simulink model "CDR_Basic_lib"  (R2012b)
settings: Solver=ode45  StartTime=0.0  StopTime=10.0  RelTol=1e-3
values from neighbouring files (symbols this model uses):
  Ts = 1/fbit/OSR    (= 0.01)    [init_pr_bb_cdr.m]
undefined symbols (not defined in the file): Fosc, Int_Divider, Tsymbol, VDD
libraries: simulink_extras x124, simulink x3
(part 1 of 2)
settings Model: ExtModeAutoUpdateStatusClock=off  Creator=Hemesh Yasotharan  LastModifiedBy=Tony
settings DataIOCC: SignalLoggingSaveFormat=ModelDataLogs
settings OptimizationCC: InitFltsAndDblsToZero=on
settings DebuggingCC: SaveWithParameterizedLinksMsg=none  FcnCallInpInsideContextMsg=UseLocalSettings  StrictBusMsg=Warning
settings GRTTargetCC: TargetFcnLib=ansi_tfl_tmw.mat  CombineOutputUpdateFcns=off  GRTInterface=on

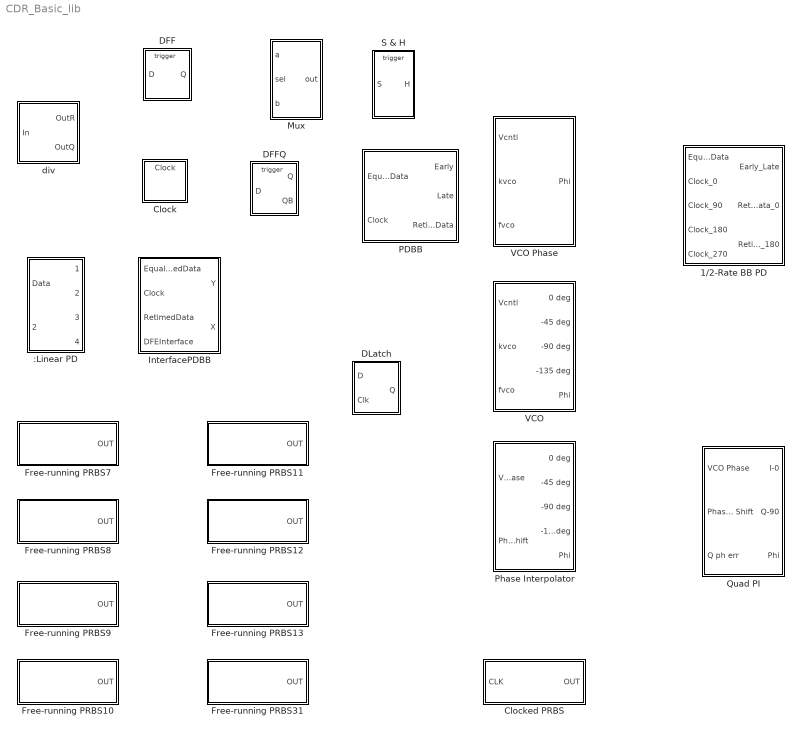
== system CDR_Basic_lib ==
  1/2-Rate BB PD : Subsystem  mask{VDD=1}
  :Linear PD : Subsystem  mask{VDD=VDD}
  Clock : Subsystem  mask{Period=0, PulseWidth=0}
      mask prompts: Period "Samples in one Period"; PulseWidth "Samples in the Pulse width"
  Clocked PRBS : Subsystem  mask{rst_time=0, X00=1, X01=1, X02=1, X03=1, X04=1, X05=1, X06=1, X07=1, X08=1, X09=1}
      mask prompts: rst_time "Reset time"; X00 "X00 [0,1]:"; X01 "X01 [0,1]:"; X02 "X02 [0,1]:"; X03 "X03 [0,1]:"; X04 "X04 [0,1]:"; X05 "X05 [0,1]:"; X06 "X06 [0,1]:"; X07 "X07 [0,1]:"; X08 "X08 [0,1]:"; X09 "X09 [0,1]:"
      mask help: Enter the initial state [0,1] below.
      mask Display: disp('PRBS_2^10')
  DFF : Subsystem  mask{DataHigh=1, DataLow=0, FF_Threshold=0.5}
      mask prompts: DataHigh "High Data Value"; DataLow "Low Data Value"; FF_Threshold "Flip-Flop Threshold"
  DFFQ : Subsystem  mask{DataHigh=1, DataLow=0, FF_Threshold=0.5}
      mask prompts: DataHigh "High Data Value"; DataLow "Low Data Value"; FF_Threshold "Flip-Flop Threshold"
  DLatch : Subsystem  mask{DataHigh=VDD, DataLow=0, L_Threshold=VDD/2}
      mask prompts: DataHigh "High Data Value"; DataLow "Low Data Value"; L_Threshold "Latch Threshold"
  Free-running PRBS10 : Subsystem  mask{sample_prd=Ts, symbol_prd=Tsymbol, X00=1, X01=1, X02=1, X03=1, X04=1, X05=1, X06=1, X07=1, X08=1, X09=1}
      mask prompts: sample_prd "Sample Time [s]:"; symbol_prd "Symbol Period [s]:"; X00 "X00 [0,1]:"; X01 "X01 [0,1]:"; X02 "X02 [0,1]:"; X03 "X03 [0,1]:"; X04 "X04 [0,1]:"; X05 "X05 [0,1]:"; X06 "X06 [0,1]:"; X07 "X07 [0,1]:"; X08 "X08 [0,1]:"; X09 "X09 [0,1]:"
      mask help: Enter the initial state [0,1] below.
      mask Display: disp('PRBS_2^10')
  Free-running PRBS11 : Subsystem  mask{sample_prd=Ts, symbol_prd=Tsymbol, X00=1, X01=1, X02=1, X03=1, X04=1, X05=1, X06=1, X07=1, X08=1, X09=1, X10=1}
      mask prompts: sample_prd "Sample Time [s]:"; symbol_prd "Symbol Period [s]:"; X00 "X00 [0,1]:"; X01 "X01 [0,1]:"; X02 "X02 [0,1]:"; X03 "X03 [0,1]:"; X04 "X04 [0,1]:"; X05 "X05 [0,1]:"; X06 "X06 [0,1]:"; X07 "X07 [0,1]:"; X08 "X08 [0,1]:"; X09 "X09 [0,1]:"; X10 "X10 [0,1]:"
      mask help: Enter the initial state [0,1] below.
      mask Display: disp('PRBS_2^11')
  Free-running PRBS12 : Subsystem  mask{sample_prd=Ts, symbol_prd=Tsymbol, X00=1, X01=1, X02=1, X03=1, X04=1, X05=1, X06=1, X07=1, X08=1, X09=1, X10=1, X11=1}
      mask prompts: sample_prd "Sample Time [s]:"; symbol_prd "Symbol Period [s]:"; X00 "X00 [0,1]:"; X01 "X01 [0,1]:"; X02 "X02 [0,1]:"; X03 "X03 [0,1]:"; X04 "X04 [0,1]:"; X05 "X05 [0,1]:"; X06 "X06 [0,1]:"; X07 "X07 [0,1]:"; X08 "X08 [0,1]:"; X09 "X09 [0,1]:"; X10 "X10 [0,1]:"; X11 "X11 [0,1]:"
      mask help: Enter the initial state [0,1] below.
      mask Display: disp('PRBS_2^12')
  Free-running PRBS13 : Subsystem  mask{sample_prd=Ts, symbol_prd=Tsymbol, X00=1, X01=1, X02=1, X03=1, X04=1, X05=1, X06=1, X07=1, X08=1, X09=1, X10=1, X11=1, X12=1}
      mask prompts: sample_prd "Sample Time [s]:"; symbol_prd "Symbol Period [s]:"; X00 "X00 [0,1]:"; X01 "X01 [0,1]:"; X02 "X02 [0,1]:"; X03 "X03 [0,1]:"; X04 "X04 [0,1]:"; X05 "X05 [0,1]:"; X06 "X06 [0,1]:"; X07 "X07 [0,1]:"; X08 "X08 [0,1]:"; X09 "X09 [0,1]:"; X10 "X10 [0,1]:"; X11 "X11 [0,1]:"; X12 "X12 [0,1]:"
      mask help: Enter the initial state [0,1] below.
      mask Display: disp('PRBS_2^13')
  Free-running PRBS31 : Subsystem  mask{sample_prd=Ts, symbol_prd=Tsymbol, X00=1, X01=1, X02=1, X03=1, X04=1, X05=1, X06=1, X07=1, X08=1, X09=1, X10=1, X11=1, X12=1, X13=1, X14=1, X15=1, X16=1, X17=1, X18=1, X19=1, X20=1, X21=1, X22=1, X23=1, X24=1, X25=1, X26=1, X27=1, X28=1, X29=1, X30=1}
      mask prompts: sample_prd "Sample Time [s]:"; symbol_prd "Symbol Period [s]:"; X00 "X00 [0,1]:"; X01 "X01 [0,1]:"; X02 "X02 [0,1]:"; X03 "X03 [0,1]:"; X04 "X04 [0,1]:"; X05 "X05 [0,1]:"; X06 "X06 [0,1]:"; X07 "X07 [0,1]:"; X08 "X08 [0,1]:"; X09 "X09 [0,1]:"; X10 "X10 [0,1]:"; X11 "X11 [0,1]:"; X12 "X12 [0,1]:"; X13 "X13 [0,1]:"; X14 "X14 [0,1]:"; X15 "X15 [0,1]:"; X16 "X16 [0,1]:"; X17 "X17 [0,1]:"; X18 "X18 [0,1]:"; X19 "X19 [0,1]:"; X20 "X20 [0,1]:"; X21 "X21 [0,1]:"; X22 "X22 [0,1]:"; X23 "X23 [0,1]:"; X24 "X24 [0,1]:"; X25 "X25 [0,1]:"; X26 "X26 [0,1]:"; X27 "X27 [0,1]:"; X28 "X28 [0,1]:"; X29 "X29 [0,1]:"; X30 "X30 [0,1]:"
      mask help: Enter the initial state [0,1] below.
      mask Display: disp('PRBS_2^31')
  Free-running PRBS7 : Subsystem  mask{sample_prd=Ts, symbol_prd=Tsymbol, X00=1, X01=1, X02=1, X03=1, X04=1, X05=1, X06=1}
      mask prompts: sample_prd "Sample Time [s]:"; symbol_prd "Symbol Period [s]:"; X00 "X00 [0,1]:"; X01 "X01 [0,1]:"; X02 "X02 [0,1]:"; X03 "X03 [0,1]:"; X04 "X04 [0,1]:"; X05 "X05 [0,1]:"; X06 "X06 [0,1]:"
      mask help: Enter the initial state [0,1] below.
      mask Display: disp('PRBS_2^7')
  Free-running PRBS8 : Subsystem  mask{sample_prd=Ts, symbol_prd=Tsymbol, X00=1, X01=1, X02=1, X03=1, X04=1, X05=1, X06=1, X07=1}
      mask prompts: sample_prd "Sample Time [s]:"; symbol_prd "Symbol Period [s]:"; X00 "X00 [0,1]:"; X01 "X01 [0,1]:"; X02 "X02 [0,1]:"; X03 "X03 [0,1]:"; X04 "X04 [0,1]:"; X05 "X05 [0,1]:"; X06 "X06 [0,1]:"; X07 "X07 [0,1]:"
      mask help: Enter the initial state [0,1] below.
      mask Display: disp('PRBS_2^8')
  Free-running PRBS9 : Subsystem  mask{sample_prd=Ts, symbol_prd=Tsymbol, X00=1, X01=1, X02=1, X03=1, X04=1, X05=1, X06=1, X07=1, X08=1}
      mask prompts: sample_prd "Sample Time [s]:"; symbol_prd "Symbol Period [s]:"; X00 "X00 [0,1]:"; X01 "X01 [0,1]:"; X02 "X02 [0,1]:"; X03 "X03 [0,1]:"; X04 "X04 [0,1]:"; X05 "X05 [0,1]:"; X06 "X06 [0,1]:"; X07 "X07 [0,1]:"; X08 "X08 [0,1]:"
      mask help: Enter the initial state [0,1] below.
      mask Display: disp('PRBS_2^9')
  InterfacePDBB : Subsystem  mask{VDD=1}
  Mux : Subsystem  mask{MuxThreshold=0.5}
      mask prompts: MuxThreshold "Threshold of Mux"
  PDBB : Subsystem  mask{VDD=1}
  Phase Interpolator : Subsystem  mask(Quad VCO){Ts=Ts}
      mask prompts: Ts "Sampling Time"
  Quad PI : Subsystem  mask(Quad VCO){Ts=Ts}
      mask prompts: Ts "Sampling Time"
  S & H : Subsystem
  VCO : Subsystem  mask(Quad VCO){po=0, fcntr=Fosc, center=0, Ts=Ts}
      mask prompts: po "Initial Phase (degrees)"; fcntr "Free Running Freq."; center "Voltage for Free-Running Freq"; Ts "Sampling Time"
      mask init:
      | ph_init = (po/360)*2*pi;
  VCO Phase : Subsystem  mask(Quad VCO){po=0, fcntr=Fosc, center=0, Ts=Ts}
      mask prompts: po "Initial Phase (degrees)"; fcntr "Free Running Freq."; center "Voltage for Free-Running Freq"; Ts "Sampling Time"
      mask init:
      | ph_init = (po/360)*2*pi;
  div : Subsystem  mask{Div_Rat=Int_Divider}
      mask prompts: Div_Rat "Divdier Ratio:"
      mask help: Frequency divider (integer multiple of 2)

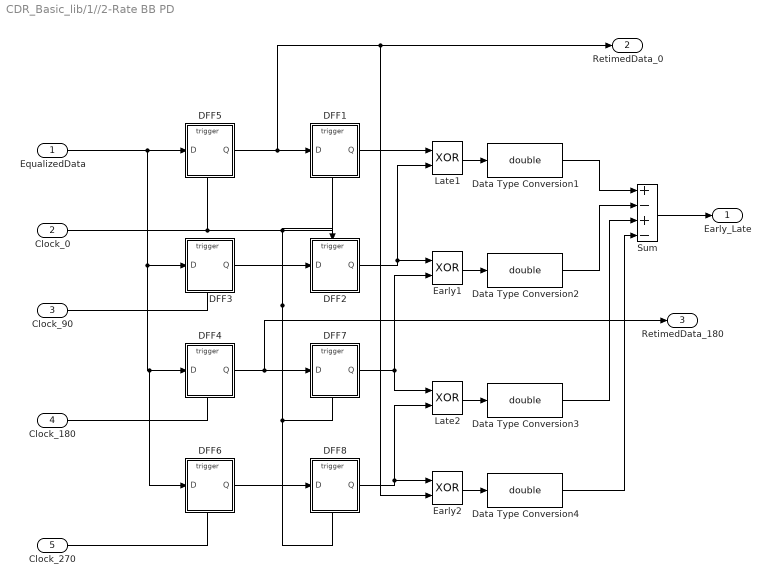
== system CDR_Basic_lib/1//2-Rate BB PD ==
  EqualizedData : Inport
  Clock_0 : Inport  Port=2
  Clock_90 : Inport  Port=3
  Clock_180 : Inport  Port=4
  Clock_270 : Inport  Port=5
  DFF1 : Subsystem  mask{DataHigh=VDD, DataLow=0, FF_Threshold=VDD/2}
      mask prompts: DataHigh "High Data Value"; DataLow "Low Data Value"; FF_Threshold "Flip-Flop Threshold"
  DFF2 : Subsystem  mask{DataHigh=VDD, DataLow=0, FF_Threshold=VDD/2}
      mask prompts: DataHigh "High Data Value"; DataLow "Low Data Value"; FF_Threshold "Flip-Flop Threshold"
  DFF3 : Subsystem  mask{DataHigh=VDD, DataLow=0, FF_Threshold=VDD/2}
      mask prompts: DataHigh "High Data Value"; DataLow "Low Data Value"; FF_Threshold "Flip-Flop Threshold"
  DFF4 : Subsystem  mask{DataHigh=VDD, DataLow=0, FF_Threshold=VDD/2}
      mask prompts: DataHigh "High Data Value"; DataLow "Low Data Value"; FF_Threshold "Flip-Flop Threshold"
  DFF5 : Subsystem  mask{DataHigh=VDD, DataLow=0, FF_Threshold=VDD/2}
      mask prompts: DataHigh "High Data Value"; DataLow "Low Data Value"; FF_Threshold "Flip-Flop Threshold"
  DFF6 : Subsystem  mask{DataHigh=VDD, DataLow=0, FF_Threshold=VDD/2}
      mask prompts: DataHigh "High Data Value"; DataLow "Low Data Value"; FF_Threshold "Flip-Flop Threshold"
  DFF7 : Subsystem  mask{DataHigh=VDD, DataLow=0, FF_Threshold=VDD/2}
      mask prompts: DataHigh "High Data Value"; DataLow "Low Data Value"; FF_Threshold "Flip-Flop Threshold"
  DFF8 : Subsystem  mask{DataHigh=VDD, DataLow=0, FF_Threshold=VDD/2}
      mask prompts: DataHigh "High Data Value"; DataLow "Low Data Value"; FF_Threshold "Flip-Flop Threshold"
  Data Type Conversion{1..4} (4 alike) : DataTypeConversion  OutDataTypeStr=double
  Early1 : Logic  Operator=XOR  AllPortsSameDT=off
  Early2 : Logic  Operator=XOR  AllPortsSameDT=off
  Late1 : Logic  Operator=XOR  AllPortsSameDT=off
  Late2 : Logic  Operator=XOR  AllPortsSameDT=off
  Sum : Sum  Inputs=+-+-
  Early_Late : Outport
  RetimedData_0 : Outport  Port=2
  RetimedData_180 : Outport  Port=3
  wires:
  EqualizedData/1 -> DFF6/1(D), DFF4/1(D), DFF3/1(D), DFF5/1(D)
  Late1/1 -> Data Type Conversion1/1
  DFF1/1(Q) -> Late1/1
  DFF2/1(Q) -> Early1/1, Late1/2
  DFF5/1(Q) -> DFF1/1(D), RetimedData_0/1, Early2/2
  DFF3/1(Q) -> DFF2/1(D)
  Clock_90/1 -> DFF3/Trigger
  Clock_180/1 -> DFF4/Trigger
  Clock_270/1 -> DFF6/Trigger
  DFF4/1(Q) -> RetimedData_180/1, DFF7/1(D)
  DFF6/1(Q) -> DFF8/1(D)
  Clock_0/1 -> DFF2/Trigger, DFF7/Trigger, DFF8/Trigger, DFF1/Trigger, DFF5/Trigger
  Early1/1 -> Data Type Conversion2/1
  DFF7/1(Q) -> Late2/1, Early1/2
  Late2/1 -> Data Type Conversion3/1
  DFF8/1(Q) -> Early2/1, Late2/2
  Early2/1 -> Data Type Conversion4/1
  Data Type Conversion1/1 -> Sum/1
  Data Type Conversion2/1 -> Sum/2
  Data Type Conversion3/1 -> Sum/3
  Data Type Conversion4/1 -> Sum/4
  Sum/1 -> Early_Late/1

== system CDR_Basic_lib/:Linear PD ==
  Data : Inport
  Clock : Inport  Port=2
  DLatch : Subsystem  mask{DataHigh=VDD, DataLow=0, L_Threshold=VDD/2}
      mask prompts: DataHigh "High Data Value"; DataLow "Low Data Value"; L_Threshold "Latch Threshold"
  DLatch1 : Subsystem  mask{DataHigh=VDD, DataLow=0, L_Threshold=VDD/2}
      mask prompts: DataHigh "High Data Value"; DataLow "Low Data Value"; L_Threshold "Latch Threshold"
  DLatch2 : Subsystem  mask{DataHigh=VDD, DataLow=0, L_Threshold=VDD/2}
      mask prompts: DataHigh "High Data Value"; DataLow "Low Data Value"; L_Threshold "Latch Threshold"
  DLatch3 : Subsystem  mask{DataHigh=VDD, DataLow=0, L_Threshold=VDD/2}
      mask prompts: DataHigh "High Data Value"; DataLow "Low Data Value"; L_Threshold "Latch Threshold"
  Data Type Conversion : DataTypeConversion  OutDataTypeStr=double
  Data Type Conversion1 : DataTypeConversion  OutDataTypeStr=double
  Logical Operator : Logic  Operator=NOT  AllPortsSameDT=off
  Logical Operator1 : Logic  Operator=XOR  AllPortsSameDT=off
  Logical Operator2 : Logic  Operator=XOR  AllPortsSameDT=off
  Error : Outport
  Reference : Outport  Port=2
  Yeven : Outport  Port=3
  Yodd : Outport  Port=4
  wires:
  DLatch3/1(Q) -> Logical Operator1/2
  DLatch1/1(Q) -> Logical Operator1/1
  DLatch2/1(Q) -> Yodd/1, DLatch3/1(D), Logical Operator2/2
  DLatch/1(Q) -> Yeven/1, DLatch1/1(D), Logical Operator2/1
  Logical Operator/1 -> DLatch1/2(Clk), DLatch2/2(Clk)
  Data/1 -> DLatch2/1(D), DLatch/1(D)
  Logical Operator2/1 -> Data Type Conversion/1
  Data Type Conversion/1 -> Error/1
  Logical Operator1/1 -> Data Type Conversion1/1
  Data Type Conversion1/1 -> Reference/1
  Clock/1 -> DLatch3/2(Clk), DLatch/2(Clk), Logical Operator/1

== system CDR_Basic_lib/Clock ==
  Constant : Constant  Value=0  SampleTime=Ts
  Pulse Generator1 : DiscretePulseGenerator  Period=Period  PulseWidth=PulseWidth  PhaseDelay=Period/2  SampleTime=Ts
  Sum2 : Sum  Inputs=|+-
  Clock : Outport
  wires:
  Sum2/1 -> Clock/1
  Pulse Generator1/1 -> Sum2/1
  Constant/1 -> Sum2/2

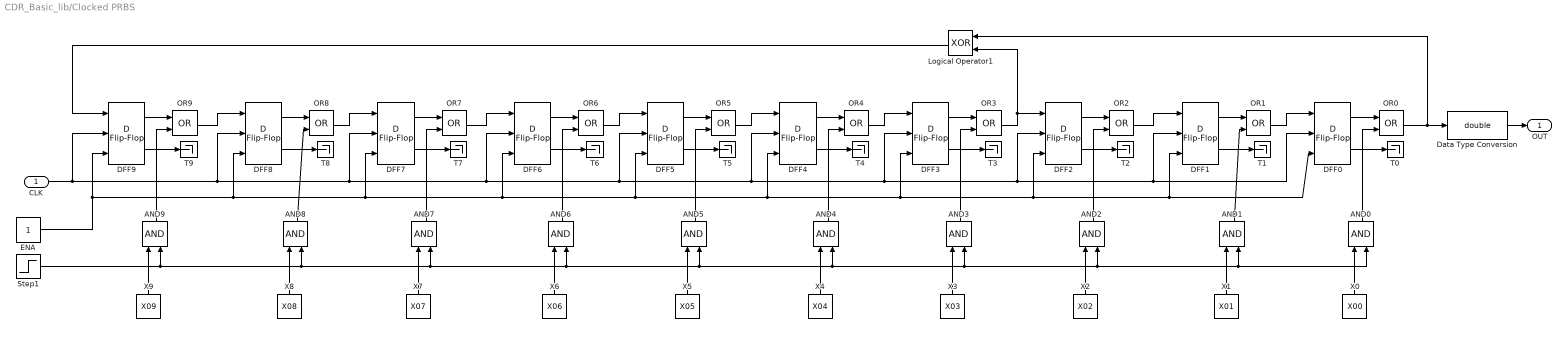
== system CDR_Basic_lib/Clocked PRBS ==
  CLK : Inport
  AND{0..9} (10 alike) : Logic  AllPortsSameDT=off  OutDataTypeStr=boolean
  DFF{0..9} (10 alike) : simulink_extras/Flip Flops/D Flip-Flop
  Data Type Conversion : DataTypeConversion  OutDataTypeStr=double
  ENA : Constant  OutDataTypeStr=boolean  SampleTime=-1
  Logical Operator1 : Logic  Operator=XOR  AllPortsSameDT=off  OutDataTypeStr=boolean
  OR{0..9} (10 alike) : Logic  Operator=OR  AllPortsSameDT=off  OutDataTypeStr=boolean
  Step1 : Step  Time=rst_time  Before=1  After=0
  T{0..9} (10 alike) : Terminator
  X0 : Constant  Value=X00  OutDataTypeStr=boolean  SampleTime=-1
  X1 : Constant  Value=X01  OutDataTypeStr=boolean  SampleTime=-1
  X2 : Constant  Value=X02  OutDataTypeStr=boolean  SampleTime=-1
  X3 : Constant  Value=X03  OutDataTypeStr=boolean  SampleTime=-1
  X4 : Constant  Value=X04  OutDataTypeStr=boolean  SampleTime=-1
  X5 : Constant  Value=X05  OutDataTypeStr=boolean  SampleTime=-1
  X6 : Constant  Value=X06  OutDataTypeStr=boolean  SampleTime=-1
  X7 : Constant  Value=X07  OutDataTypeStr=boolean  SampleTime=-1
  X8 : Constant  Value=X08  OutDataTypeStr=boolean  SampleTime=-1
  X9 : Constant  Value=X09  OutDataTypeStr=boolean  SampleTime=-1
  OUT : Outport
  wires:
  AND6/1 -> OR6/2
  AND5/1 -> OR5/2
  AND4/1 -> OR4/2
  AND3/1 -> OR3/2
  AND2/1 -> OR2/2
  AND0/1 -> OR0/2
  AND1/1 -> OR1/2
  OR0/1 -> Logical Operator1/1, Data Type Conversion/1
  OR1/1 -> DFF0/1
  DFF0/2 -> T0/1
  DFF0/1 -> OR0/1
  OR2/1 -> DFF1/1
  DFF1/2 -> T1/1
  DFF1/1 -> OR1/1
  OR3/1 -> DFF2/1, Logical Operator1/2
  DFF2/2 -> T2/1
  DFF2/1 -> OR2/1
  OR4/1 -> DFF3/1
  DFF3/2 -> T3/1
  DFF3/1 -> OR3/1
  OR5/1 -> DFF4/1
  DFF4/2 -> T4/1
  DFF4/1 -> OR4/1
  OR6/1 -> DFF5/1
  DFF5/2 -> T5/1
  DFF5/1 -> OR5/1
  DFF6/2 -> T6/1
  DFF6/1 -> OR6/1
  X6/1 -> AND6/1
  X1/1 -> AND1/1
  X3/1 -> AND3/1
  X4/1 -> AND4/1
  X5/1 -> AND5/1
  X0/1 -> AND0/1
  X2/1 -> AND2/1
  AND9/1 -> OR9/2
  AND7/1 -> OR7/2
  AND8/1 -> OR8/2
  OR8/1 -> DFF7/1
  DFF7/2 -> T7/1
  DFF7/1 -> OR7/1
  OR9/1 -> DFF8/1
  DFF8/2 -> T8/1
  DFF8/1 -> OR8/1
  DFF9/2 -> T9/1
  DFF9/1 -> OR9/1
  X8/1 -> AND8/1
  X7/1 -> AND7/1
  X9/1 -> AND9/1
  OR7/1 -> DFF6/1
  CLK/1 -> DFF9/2, DFF8/2, DFF7/2, DFF6/2, DFF5/2, DFF0/2, DFF1/2, DFF2/2, DFF3/2, DFF4/2
  ENA/1 -> DFF9/3, DFF8/3, DFF7/3, DFF6/3, DFF4/3, DFF0/3, DFF1/3, DFF2/3, DFF3/3, DFF5/3
  Logical Operator1/1 -> DFF9/1
  Step1/1 -> AND9/2, AND8/2, AND7/2, AND5/2, AND0/2, AND1/2, AND2/2, AND3/2, AND4/2, AND6/2
  Data Type Conversion/1 -> OUT/1

== system CDR_Basic_lib/DFF ==
  D : Inport  LatchByDelayingOutsideSignal=on
  Trigger : TriggerPort
  High Value : Constant  Value=DataHigh
  Low Value : Constant  Value=DataLow
  Switch : Switch  Threshold=FF_Threshold
  Q : Outport
  wires:
  Low Value/1 -> Switch/3
  High Value/1 -> Switch/1
  D/1 -> Switch/2
  Switch/1 -> Q/1

== system CDR_Basic_lib/DFFQ ==
  D : Inport  LatchByDelayingOutsideSignal=on
  Trigger : TriggerPort
  High Value : Constant  Value=DataHigh
  Logical Operator : Logic  Operator=NOT  AllPortsSameDT=off  OutDataTypeStr=boolean
  Low Value : Constant  Value=DataLow
  Switch : Switch  Threshold=FF_Threshold
  Q : Outport
  QB : Outport  Port=2
  wires:
  Low Value/1 -> Switch/3
  High Value/1 -> Switch/1
  D/1 -> Switch/2
  Switch/1 -> Q/1, Logical Operator/1
  Logical Operator/1 -> QB/1

== system CDR_Basic_lib/DLatch ==
  D : Inport
  Clk : Inport  Port=2
  Constant : Constant  Value=L_Threshold
  D Latch : simulink_extras/Flip Flops/D Latch  SystemSampleTime=-1
  Data Type Conversion1 : DataTypeConversion  OutDataTypeStr=boolean
  Data Type Conversion2 : DataTypeConversion  OutDataTypeStr=double
  Data Type Conversion3 : DataTypeConversion  OutDataTypeStr=double
  Gain : Gain  Gain=DataHigh
  Gain1 : Gain  Gain=DataHigh
  Relational Operator : RelationalOperator  OutDataTypeStr=boolean
  Q : Outport
  wires:
  D/1 -> Relational Operator/1
  Clk/1 -> Data Type Conversion1/1
  Data Type Conversion1/1 -> D Latch/2
  D Latch/1 -> Data Type Conversion2/1
  D Latch/2 -> Data Type Conversion3/1
  Data Type Conversion2/1 -> Gain/1
  Gain/1 -> Q/1
  Data Type Conversion3/1 -> Gain1/1
  Relational Operator/1 -> D Latch/1
  Constant/1 -> Relational Operator/2

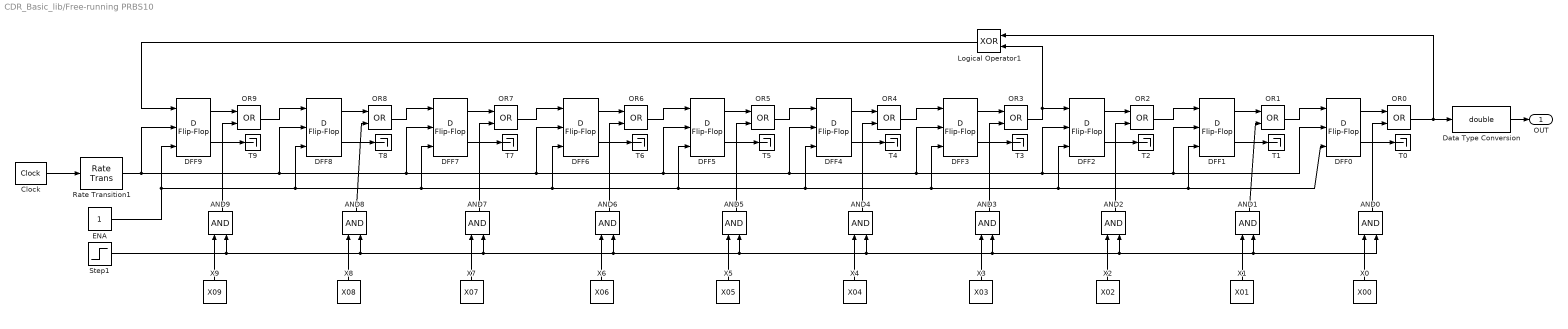
== system CDR_Basic_lib/Free-running PRBS10 ==
  AND{0..9} (10 alike) : Logic  AllPortsSameDT=off  OutDataTypeStr=boolean
  Clock : simulink_extras/Flip Flops/Clock  period=symbol_prd
  DFF{0..9} (10 alike) : simulink_extras/Flip Flops/D Flip-Flop
  Data Type Conversion : DataTypeConversion  OutDataTypeStr=double
  ENA : Constant  OutDataTypeStr=boolean  SampleTime=sample_prd
  Logical Operator1 : Logic  Operator=XOR  AllPortsSameDT=off  OutDataTypeStr=boolean
  OR{0..9} (10 alike) : Logic  Operator=OR  AllPortsSameDT=off  OutDataTypeStr=boolean
  Rate Transition1 : RateTransition  OutPortSampleTime=sample_prd
  Step1 : Step  Time=symbol_prd  Before=1  After=0  SampleTime=sample_prd
  T{0..9} (10 alike) : Terminator
  X0 : Constant  Value=X00  OutDataTypeStr=boolean  SampleTime=sample_prd
  X1 : Constant  Value=X01  OutDataTypeStr=boolean  SampleTime=sample_prd
  X2 : Constant  Value=X02  OutDataTypeStr=boolean  SampleTime=sample_prd
  X3 : Constant  Value=X03  OutDataTypeStr=boolean  SampleTime=sample_prd
  X4 : Constant  Value=X04  OutDataTypeStr=boolean  SampleTime=sample_prd
  X5 : Constant  Value=X05  OutDataTypeStr=boolean  SampleTime=sample_prd
  X6 : Constant  Value=X06  OutDataTypeStr=boolean  SampleTime=sample_prd
  X7 : Constant  Value=X07  OutDataTypeStr=boolean  SampleTime=sample_prd
  X8 : Constant  Value=X08  OutDataTypeStr=boolean  SampleTime=sample_prd
  X9 : Constant  Value=X09  OutDataTypeStr=boolean  SampleTime=sample_prd
  OUT : Outport
  wires:
  Data Type Conversion/1 -> OUT/1
  Step1/1 -> AND6/2, AND4/2, AND3/2, AND2/2, AND1/2, AND0/2, AND5/2, AND7/2, AND8/2, AND9/2
  Logical Operator1/1 -> DFF9/1
  ENA/1 -> DFF5/3, DFF3/3, DFF2/3, DFF1/3, DFF0/3, DFF4/3, DFF6/3, DFF7/3, DFF8/3, DFF9/3
  Rate Transition1/1 -> DFF4/2, DFF3/2, DFF2/2, DFF1/2, DFF0/2, DFF5/2, DFF6/2, DFF7/2, DFF8/2, DFF9/2
  OR7/1 -> DFF6/1
  Clock/1 -> Rate Transition1/1
  X9/1 -> AND9/1
  X7/1 -> AND7/1
  X8/1 -> AND8/1
  DFF9/1 -> OR9/1
  DFF9/2 -> T9/1
  DFF8/1 -> OR8/1
  DFF8/2 -> T8/1
  OR9/1 -> DFF8/1
  DFF7/1 -> OR7/1
  DFF7/2 -> T7/1
  OR8/1 -> DFF7/1
  AND8/1 -> OR8/2
  AND7/1 -> OR7/2
  AND9/1 -> OR9/2
  X2/1 -> AND2/1
  X0/1 -> AND0/1
  X5/1 -> AND5/1
  X4/1 -> AND4/1
  X3/1 -> AND3/1
  X1/1 -> AND1/1
  X6/1 -> AND6/1
  DFF6/1 -> OR6/1
  DFF6/2 -> T6/1
  DFF5/1 -> OR5/1
  DFF5/2 -> T5/1
  OR6/1 -> DFF5/1
  DFF4/1 -> OR4/1
  DFF4/2 -> T4/1
  OR5/1 -> DFF4/1
  DFF3/1 -> OR3/1
  DFF3/2 -> T3/1
  OR4/1 -> DFF3/1
  DFF2/1 -> OR2/1
  DFF2/2 -> T2/1
  OR3/1 -> Logical Operator1/2, DFF2/1
  DFF1/1 -> OR1/1
  DFF1/2 -> T1/1
  OR2/1 -> DFF1/1
  DFF0/1 -> OR0/1
  DFF0/2 -> T0/1
  OR1/1 -> DFF0/1
  OR0/1 -> Data Type Conversion/1, Logical Operator1/1
  AND1/1 -> OR1/2
  AND0/1 -> OR0/2
  AND2/1 -> OR2/2
  AND3/1 -> OR3/2
  AND4/1 -> OR4/2
  AND5/1 -> OR5/2
  AND6/1 -> OR6/2

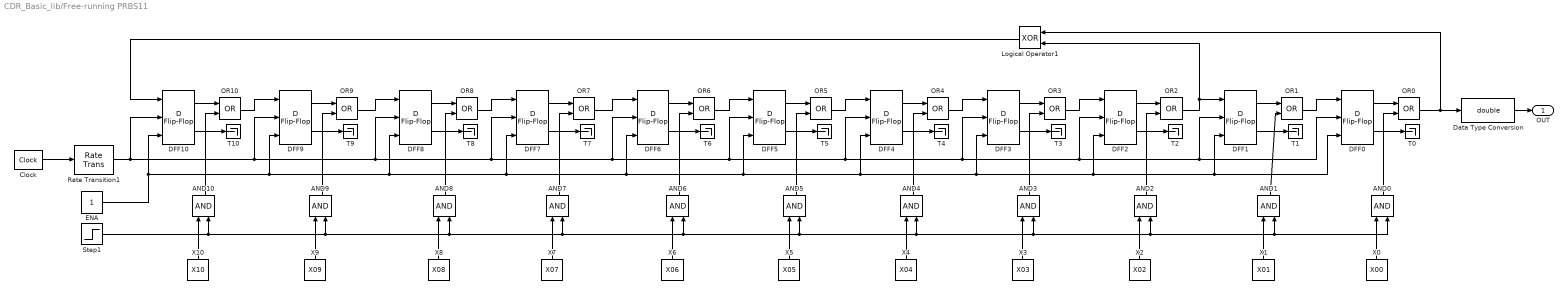
== system CDR_Basic_lib/Free-running PRBS11 ==
  AND{0..10} (11 alike) : Logic  AllPortsSameDT=off  OutDataTypeStr=boolean
  Clock : simulink_extras/Flip Flops/Clock  period=symbol_prd
  DFF{0..10} (11 alike) : simulink_extras/Flip Flops/D Flip-Flop
  Data Type Conversion : DataTypeConversion  OutDataTypeStr=double
  ENA : Constant  OutDataTypeStr=boolean  SampleTime=sample_prd
  Logical Operator1 : Logic  Operator=XOR  AllPortsSameDT=off  OutDataTypeStr=boolean
  OR{0..10} (11 alike) : Logic  Operator=OR  AllPortsSameDT=off  OutDataTypeStr=boolean
  Rate Transition1 : RateTransition  OutPortSampleTime=sample_prd
  Step1 : Step  Time=symbol_prd  Before=1  After=0  SampleTime=sample_prd
  T{0..10} (11 alike) : Terminator
  X0 : Constant  Value=X00  OutDataTypeStr=boolean  SampleTime=sample_prd
  X1 : Constant  Value=X01  OutDataTypeStr=boolean  SampleTime=sample_prd
  X10 : Constant  Value=X10  OutDataTypeStr=boolean  SampleTime=sample_prd
  X2 : Constant  Value=X02  OutDataTypeStr=boolean  SampleTime=sample_prd
  X3 : Constant  Value=X03  OutDataTypeStr=boolean  SampleTime=sample_prd
  X4 : Constant  Value=X04  OutDataTypeStr=boolean  SampleTime=sample_prd
  X5 : Constant  Value=X05  OutDataTypeStr=boolean  SampleTime=sample_prd
  X6 : Constant  Value=X06  OutDataTypeStr=boolean  SampleTime=sample_prd
  X7 : Constant  Value=X07  OutDataTypeStr=boolean  SampleTime=sample_prd
  X8 : Constant  Value=X08  OutDataTypeStr=boolean  SampleTime=sample_prd
  X9 : Constant  Value=X09  OutDataTypeStr=boolean  SampleTime=sample_prd
  OUT : Outport
  wires:
  Data Type Conversion/1 -> OUT/1
  Step1/1 -> AND2/2, AND1/2, AND0/2, AND3/2, AND4/2, AND5/2, AND6/2, AND7/2, AND8/2, AND9/2, AND10/2
  Logical Operator1/1 -> DFF10/1
  ENA/1 -> DFF6/3, DFF5/3, DFF4/3, DFF3/3, DFF2/3, DFF1/3, DFF0/3, DFF7/3, DFF8/3, DFF9/3, DFF10/3
  Rate Transition1/1 -> DFF8/2, DFF5/2, DFF4/2, DFF3/2, DFF2/2, DFF1/2, DFF0/2, DFF6/2, DFF7/2, DFF9/2, DFF10/2
  OR7/1 -> DFF6/1
  Clock/1 -> Rate Transition1/1
  X9/1 -> AND9/1
  X7/1 -> AND7/1
  X10/1 -> AND10/1
  X8/1 -> AND8/1
  DFF10/1 -> OR10/1
  DFF10/2 -> T10/1
  DFF9/1 -> OR9/1
  DFF9/2 -> T9/1
  OR10/1 -> DFF9/1
  DFF8/1 -> OR8/1
  DFF8/2 -> T8/1
  OR9/1 -> DFF8/1
  DFF7/1 -> OR7/1
  DFF7/2 -> T7/1
  OR8/1 -> DFF7/1
  AND8/1 -> OR8/2
  AND7/1 -> OR7/2
  AND9/1 -> OR9/2
  AND10/1 -> OR10/2
  X2/1 -> AND2/1
  X0/1 -> AND0/1
  X5/1 -> AND5/1
  X4/1 -> AND4/1
  X3/1 -> AND3/1
  X1/1 -> AND1/1
  X6/1 -> AND6/1
  DFF6/1 -> OR6/1
  DFF6/2 -> T6/1
  DFF5/1 -> OR5/1
  DFF5/2 -> T5/1
  OR6/1 -> DFF5/1
  DFF4/1 -> OR4/1
  DFF4/2 -> T4/1
  OR5/1 -> DFF4/1
  DFF3/1 -> OR3/1
  DFF3/2 -> T3/1
  OR4/1 -> DFF3/1
  DFF2/1 -> OR2/1
  DFF2/2 -> T2/1
  OR3/1 -> DFF2/1
  DFF1/1 -> OR1/1
  DFF1/2 -> T1/1
  OR2/1 -> Logical Operator1/2, DFF1/1
  DFF0/1 -> OR0/1
  DFF0/2 -> T0/1
  OR1/1 -> DFF0/1
  OR0/1 -> Data Type Conversion/1, Logical Operator1/1
  AND1/1 -> OR1/2
  AND0/1 -> OR0/2
  AND2/1 -> OR2/2
  AND3/1 -> OR3/2
  AND4/1 -> OR4/2
  AND5/1 -> OR5/2
  AND6/1 -> OR6/2

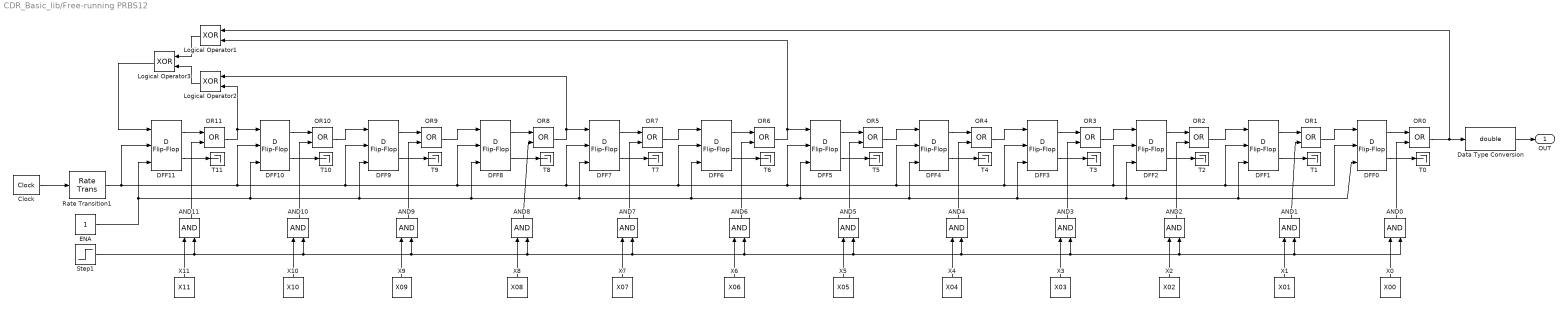
== system CDR_Basic_lib/Free-running PRBS12 ==
  AND{0..11} (12 alike) : Logic  AllPortsSameDT=off  OutDataTypeStr=boolean
  Clock : simulink_extras/Flip Flops/Clock  period=symbol_prd
  DFF{0..11} (12 alike) : simulink_extras/Flip Flops/D Flip-Flop
  Data Type Conversion : DataTypeConversion  OutDataTypeStr=double
  ENA : Constant  OutDataTypeStr=boolean  SampleTime=sample_prd
  Logical Operator1 : Logic  Operator=XOR  AllPortsSameDT=off  OutDataTypeStr=boolean
  Logical Operator2 : Logic  Operator=XOR  AllPortsSameDT=off  OutDataTypeStr=boolean
  Logical Operator3 : Logic  Operator=XOR  AllPortsSameDT=off  OutDataTypeStr=boolean
  OR{0..11} (12 alike) : Logic  Operator=OR  AllPortsSameDT=off  OutDataTypeStr=boolean
  Rate Transition1 : RateTransition  OutPortSampleTime=sample_prd
  Step1 : Step  Time=symbol_prd  Before=1  After=0  SampleTime=sample_prd
  T{0..11} (12 alike) : Terminator
  X0 : Constant  Value=X00  OutDataTypeStr=boolean  SampleTime=sample_prd
  X1 : Constant  Value=X01  OutDataTypeStr=boolean  SampleTime=sample_prd
  X10 : Constant  Value=X10  OutDataTypeStr=boolean  SampleTime=sample_prd
  X11 : Constant  Value=X11  OutDataTypeStr=boolean  SampleTime=sample_prd
  X2 : Constant  Value=X02  OutDataTypeStr=boolean  SampleTime=sample_prd
  X3 : Constant  Value=X03  OutDataTypeStr=boolean  SampleTime=sample_prd
  X4 : Constant  Value=X04  OutDataTypeStr=boolean  SampleTime=sample_prd
  X5 : Constant  Value=X05  OutDataTypeStr=boolean  SampleTime=sample_prd
  X6 : Constant  Value=X06  OutDataTypeStr=boolean  SampleTime=sample_prd
  X7 : Constant  Value=X07  OutDataTypeStr=boolean  SampleTime=sample_prd
  X8 : Constant  Value=X08  OutDataTypeStr=boolean  SampleTime=sample_prd
  X9 : Constant  Value=X09  OutDataTypeStr=boolean  SampleTime=sample_prd
  OUT : Outport
  wires:
  Data Type Conversion/1 -> OUT/1
  Step1/1 -> AND5/2, AND1/2, AND0/2, AND2/2, AND3/2, AND4/2, AND6/2, AND7/2, AND8/2, AND9/2, AND10/2, AND11/2
  Logical Operator3/1 -> DFF11/1
  Logical Operator2/1 -> Logical Operator3/2
  Logical Operator1/1 -> Logical Operator3/1
  ENA/1 -> DFF5/3, DFF4/3, DFF3/3, DFF2/3, DFF1/3, DFF0/3, DFF6/3, DFF7/3, DFF8/3, DFF9/3, DFF10/3, DFF11/3
  Rate Transition1/1 -> DFF8/2, DFF5/2, DFF4/2, DFF2/2, DFF1/2, DFF0/2, DFF3/2, DFF6/2, DFF7/2, DFF9/2, DFF10/2, DFF11/2
  OR7/1 -> DFF6/1
  Clock/1 -> Rate Transition1/1
  X9/1 -> AND9/1
  X7/1 -> AND7/1
  X11/1 -> AND11/1
  X10/1 -> AND10/1
  X8/1 -> AND8/1
  DFF11/1 -> OR11/1
  DFF11/2 -> T11/1
  DFF10/1 -> OR10/1
  DFF10/2 -> T10/1
  OR11/1 -> Logical Operator2/2, DFF10/1
  DFF9/1 -> OR9/1
  DFF9/2 -> T9/1
  OR10/1 -> DFF9/1
  DFF8/1 -> OR8/1
  DFF8/2 -> T8/1
  OR9/1 -> DFF8/1
  DFF7/1 -> OR7/1
  DFF7/2 -> T7/1
  OR8/1 -> Logical Operator2/1, DFF7/1
  AND8/1 -> OR8/2
  AND7/1 -> OR7/2
  AND9/1 -> OR9/2
  AND10/1 -> OR10/2
  AND11/1 -> OR11/2
  X2/1 -> AND2/1
  X0/1 -> AND0/1
  X5/1 -> AND5/1
  X4/1 -> AND4/1
  X3/1 -> AND3/1
  X1/1 -> AND1/1
  X6/1 -> AND6/1
  DFF6/1 -> OR6/1
  DFF6/2 -> T6/1
  DFF5/1 -> OR5/1
  DFF5/2 -> T5/1
  OR6/1 -> Logical Operator1/2, DFF5/1
  DFF4/1 -> OR4/1
  DFF4/2 -> T4/1
  OR5/1 -> DFF4/1
  DFF3/1 -> OR3/1
  DFF3/2 -> T3/1
  OR4/1 -> DFF3/1
  DFF2/1 -> OR2/1
  DFF2/2 -> T2/1
  OR3/1 -> DFF2/1
  DFF1/1 -> OR1/1
  DFF1/2 -> T1/1
  OR2/1 -> DFF1/1
  DFF0/1 -> OR0/1
  DFF0/2 -> T0/1
  OR1/1 -> DFF0/1
  OR0/1 -> Data Type Conversion/1, Logical Operator1/1
  AND1/1 -> OR1/2
  AND0/1 -> OR0/2
  AND2/1 -> OR2/2
  AND3/1 -> OR3/2
  AND4/1 -> OR4/2
  AND5/1 -> OR5/2
  AND6/1 -> OR6/2

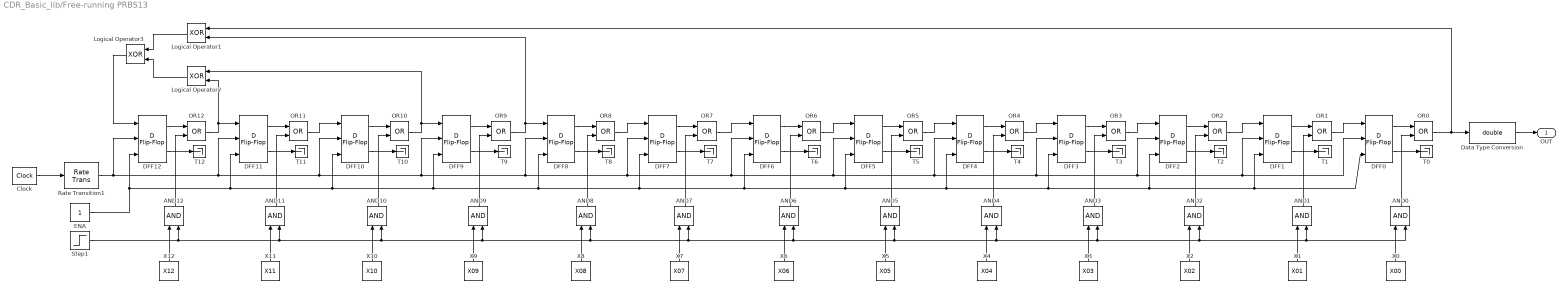
== system CDR_Basic_lib/Free-running PRBS13 ==
  AND{0..12} (13 alike) : Logic  AllPortsSameDT=off  OutDataTypeStr=boolean
  Clock : simulink_extras/Flip Flops/Clock  period=symbol_prd
  DFF{0..12} (13 alike) : simulink_extras/Flip Flops/D Flip-Flop
  Data Type Conversion : DataTypeConversion  OutDataTypeStr=double
  ENA : Constant  OutDataTypeStr=boolean  SampleTime=sample_prd
  Logical Operator1 : Logic  Operator=XOR  AllPortsSameDT=off  OutDataTypeStr=boolean
  Logical Operator2 : Logic  Operator=XOR  AllPortsSameDT=off  OutDataTypeStr=boolean
  Logical Operator3 : Logic  Operator=XOR  AllPortsSameDT=off  OutDataTypeStr=boolean
  OR{0..12} (13 alike) : Logic  Operator=OR  AllPortsSameDT=off  OutDataTypeStr=boolean
  Rate Transition1 : RateTransition  OutPortSampleTime=sample_prd
  Step1 : Step  Time=symbol_prd  Before=1  After=0  SampleTime=sample_prd
  T{0..12} (13 alike) : Terminator
  X0 : Constant  Value=X00  OutDataTypeStr=boolean  SampleTime=sample_prd
  X1 : Constant  Value=X01  OutDataTypeStr=boolean  SampleTime=sample_prd
  X10 : Constant  Value=X10  OutDataTypeStr=boolean  SampleTime=sample_prd
  X11 : Constant  Value=X11  OutDataTypeStr=boolean  SampleTime=sample_prd
  X12 : Constant  Value=X12  OutDataTypeStr=boolean  SampleTime=sample_prd
  X2 : Constant  Value=X02  OutDataTypeStr=boolean  SampleTime=sample_prd
  X3 : Constant  Value=X03  OutDataTypeStr=boolean  SampleTime=sample_prd
  X4 : Constant  Value=X04  OutDataTypeStr=boolean  SampleTime=sample_prd
  X5 : Constant  Value=X05  OutDataTypeStr=boolean  SampleTime=sample_prd
  X6 : Constant  Value=X06  OutDataTypeStr=boolean  SampleTime=sample_prd
  X7 : Constant  Value=X07  OutDataTypeStr=boolean  SampleTime=sample_prd
  X8 : Constant  Value=X08  OutDataTypeStr=boolean  SampleTime=sample_prd
  X9 : Constant  Value=X09  OutDataTypeStr=boolean  SampleTime=sample_prd
  OUT : Outport
  wires:
  Data Type Conversion/1 -> OUT/1
  Logical Operator2/1 -> Logical Operator3/2
  Logical Operator1/1 -> Logical Operator3/1
  Logical Operator3/1 -> DFF12/1
  Step1/1 -> AND12/2, AND6/2, AND5/2, AND4/2, AND3/2, AND1/2, AND0/2, AND2/2, AND7/2, AND8/2, AND9/2, AND10/2, AND11/2
  ENA/1 -> DFF7/3, DFF4/3, DFF3/3, DFF1/3, DFF0/3, DFF2/3, DFF5/3, DFF6/3, DFF8/3, DFF9/3, DFF10/3, DFF11/3, DFF12/3
  Rate Transition1/1 -> DFF9/2, DFF7/2, DFF5/2, DFF4/2, DFF3/2, DFF2/2, DFF1/2, DFF0/2, DFF6/2, DFF8/2, DFF10/2, DFF11/2, DFF12/2
  OR7/1 -> DFF6/1
  Clock/1 -> Rate Transition1/1
  X9/1 -> AND9/1
  X7/1 -> AND7/1
  X12/1 -> AND12/1
  X11/1 -> AND11/1
  X10/1 -> AND10/1
  X8/1 -> AND8/1
  DFF12/1 -> OR12/1
  DFF12/2 -> T12/1
  DFF11/1 -> OR11/1
  DFF11/2 -> T11/1
  OR12/1 -> Logical Operator2/2, DFF11/1
  DFF10/1 -> OR10/1
  DFF10/2 -> T10/1
  OR11/1 -> DFF10/1
  DFF9/1 -> OR9/1
  DFF9/2 -> T9/1
  OR10/1 -> Logical Operator2/1, DFF9/1
  DFF8/1 -> OR8/1
  DFF8/2 -> T8/1
  OR9/1 -> Logical Operator1/2, DFF8/1
  DFF7/1 -> OR7/1
  DFF7/2 -> T7/1
  OR8/1 -> DFF7/1
  AND8/1 -> OR8/2
  AND7/1 -> OR7/2
  AND9/1 -> OR9/2
  AND10/1 -> OR10/2
  AND11/1 -> OR11/2
  AND12/1 -> OR12/2
  X2/1 -> AND2/1
  X0/1 -> AND0/1
  X5/1 -> AND5/1
  X4/1 -> AND4/1
  X3/1 -> AND3/1
  X1/1 -> AND1/1
  X6/1 -> AND6/1
  DFF6/1 -> OR6/1
  DFF6/2 -> T6/1
  DFF5/1 -> OR5/1
  DFF5/2 -> T5/1
  OR6/1 -> DFF5/1
  DFF4/1 -> OR4/1
  DFF4/2 -> T4/1
  OR5/1 -> DFF4/1
  DFF3/1 -> OR3/1
  DFF3/2 -> T3/1
  OR4/1 -> DFF3/1
  DFF2/1 -> OR2/1
  DFF2/2 -> T2/1
  OR3/1 -> DFF2/1
  DFF1/1 -> OR1/1
  DFF1/2 -> T1/1
  OR2/1 -> DFF1/1
  DFF0/1 -> OR0/1
  DFF0/2 -> T0/1
  OR1/1 -> DFF0/1
  OR0/1 -> Data Type Conversion/1, Logical Operator1/1
  AND1/1 -> OR1/2
  AND0/1 -> OR0/2
  AND2/1 -> OR2/2
  AND3/1 -> OR3/2
  AND4/1 -> OR4/2
  AND5/1 -> OR5/2
  AND6/1 -> OR6/2

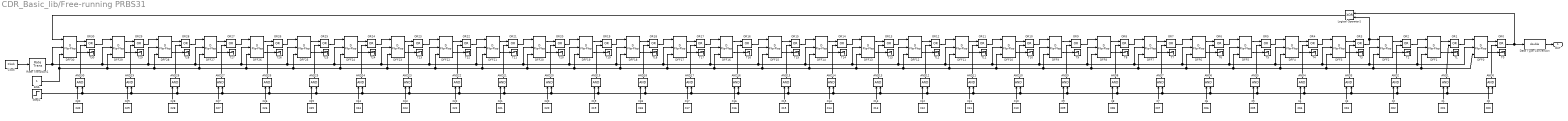
== system CDR_Basic_lib/Free-running PRBS31 ==
  AND{0..30} (31 alike) : Logic  AllPortsSameDT=off  OutDataTypeStr=boolean
  Clock : simulink_extras/Flip Flops/Clock  period=symbol_prd
  DFF{0..30} (31 alike) : simulink_extras/Flip Flops/D Flip-Flop
  Data Type Conversion : DataTypeConversion  OutDataTypeStr=double
  ENA : Constant  OutDataTypeStr=boolean  SampleTime=sample_prd
  Logical Operator1 : Logic  Operator=XOR  AllPortsSameDT=off  OutDataTypeStr=boolean
  OR{0..30} (31 alike) : Logic  Operator=OR  AllPortsSameDT=off  OutDataTypeStr=boolean
  Rate Transition1 : RateTransition  OutPortSampleTime=sample_prd
  Step1 : Step  Time=symbol_prd  Before=1  After=0  SampleTime=sample_prd
  T{0..30} (31 alike) : Terminator
  X0 : Constant  Value=X00  OutDataTypeStr=boolean  SampleTime=sample_prd
  X1 : Constant  Value=X01  OutDataTypeStr=boolean  SampleTime=sample_prd
  X10 : Constant  Value=X10  OutDataTypeStr=boolean  SampleTime=sample_prd
  X11 : Constant  Value=X11  OutDataTypeStr=boolean  SampleTime=sample_prd
  X12 : Constant  Value=X12  OutDataTypeStr=boolean  SampleTime=sample_prd
  X13 : Constant  Value=X13  OutDataTypeStr=boolean  SampleTime=sample_prd
  X14 : Constant  Value=X14  OutDataTypeStr=boolean  SampleTime=sample_prd
  X15 : Constant  Value=X15  OutDataTypeStr=boolean  SampleTime=sample_prd
  X16 : Constant  Value=X16  OutDataTypeStr=boolean  SampleTime=sample_prd
  X17 : Constant  Value=X17  OutDataTypeStr=boolean  SampleTime=sample_prd
  X18 : Constant  Value=X18  OutDataTypeStr=boolean  SampleTime=sample_prd
  X19 : Constant  Value=X19  OutDataTypeStr=boolean  SampleTime=sample_prd
  X2 : Constant  Value=X02  OutDataTypeStr=boolean  SampleTime=sample_prd
  X20 : Constant  Value=X20  OutDataTypeStr=boolean  SampleTime=sample_prd
  X21 : Constant  Value=X21  OutDataTypeStr=boolean  SampleTime=sample_prd
  X22 : Constant  Value=X22  OutDataTypeStr=boolean  SampleTime=sample_prd
  X23 : Constant  Value=X23  OutDataTypeStr=boolean  SampleTime=sample_prd
  X24 : Constant  Value=X24  OutDataTypeStr=boolean  SampleTime=sample_prd
  X25 : Constant  Value=X25  OutDataTypeStr=boolean  SampleTime=sample_prd
  X26 : Constant  Value=X26  OutDataTypeStr=boolean  SampleTime=sample_prd
  X27 : Constant  Value=X27  OutDataTypeStr=boolean  SampleTime=sample_prd
  X28 : Constant  Value=X28  OutDataTypeStr=boolean  SampleTime=sample_prd
  X29 : Constant  Value=X29  OutDataTypeStr=boolean  SampleTime=sample_prd
  X3 : Constant  Value=X03  OutDataTypeStr=boolean  SampleTime=sample_prd
  X30 : Constant  Value=X30  OutDataTypeStr=boolean  SampleTime=sample_prd
  X4 : Constant  Value=X04  OutDataTypeStr=boolean  SampleTime=sample_prd
  X5 : Constant  Value=X05  OutDataTypeStr=boolean  SampleTime=sample_prd
  X6 : Constant  Value=X06  OutDataTypeStr=boolean  SampleTime=sample_prd
  X7 : Constant  Value=X07  OutDataTypeStr=boolean  SampleTime=sample_prd
  X8 : Constant  Value=X08  OutDataTypeStr=boolean  SampleTime=sample_prd
  X9 : Constant  Value=X09  OutDataTypeStr=boolean  SampleTime=sample_prd
  OUT : Outport
  wires:
  Data Type Conversion/1 -> OUT/1
  Logical Operator1/1 -> DFF30/1
  ENA/1 -> DFF28/3, DFF26/3, DFF19/3, DFF12/3, DFF5/3, DFF3/3, DFF0/3, DFF1/3, DFF2/3, DFF4/3, DFF6/3, DFF7/3, DFF8/3, DFF9/3, DFF10/3, DFF11/3, DFF13/3, DFF14/3, DFF15/3, DFF16/3, DFF17/3, DFF18/3, DFF20/3, DFF21/3, DFF22/3, DFF23/3, DFF24/3, DFF25/3, DFF27/3, DFF29/3, DFF30/3
  Rate Transition1/1 -> DFF28/2, DFF27/2, DFF26/2, DFF24/2, DFF23/2, DFF20/2, DFF19/2, DFF17/2, DFF16/2, DFF13/2, DFF12/2, DFF10/2, DFF9/2, DFF6/2, DFF5/2, DFF3/2, DFF2/2, DFF1/2, DFF0/2, DFF4/2, DFF7/2, DFF8/2, DFF11/2, DFF14/2, DFF15/2, DFF18/2, DFF21/2, DFF22/2, DFF25/2, DFF29/2, DFF30/2
  OR7/1 -> DFF6/1
  OR14/1 -> DFF13/1
  OR21/1 -> DFF20/1
  OR28/1 -> DFF27/1
  Step1/1 -> AND28/2, AND0/2, AND1/2, AND2/2, AND3/2, AND4/2, AND5/2, AND6/2, AND7/2, AND8/2, AND9/2, AND10/2, AND11/2, AND12/2, AND13/2, AND14/2, AND15/2, AND16/2, AND17/2, AND18/2, AND19/2, AND20/2, AND21/2, AND22/2, AND23/2, AND24/2, AND25/2, AND26/2, AND27/2, AND29/2, AND30/2
  Clock/1 -> Rate Transition1/1
  X30/1 -> AND30/1
  X28/1 -> AND28/1
  X29/1 -> AND29/1
  DFF30/1 -> OR30/1
  DFF30/2 -> T30/1
  DFF29/1 -> OR29/1
  DFF29/2 -> T29/1
  OR30/1 -> DFF29/1
  DFF28/1 -> OR28/1
  DFF28/2 -> T28/1
  OR29/1 -> DFF28/1
  AND29/1 -> OR29/2
  AND28/1 -> OR28/2
  AND30/1 -> OR30/2
  X23/1 -> AND23/1
  X21/1 -> AND21/1
  X26/1 -> AND26/1
  X25/1 -> AND25/1
  X24/1 -> AND24/1
  X22/1 -> AND22/1
  X27/1 -> AND27/1
  DFF27/1 -> OR27/1
  DFF27/2 -> T27/1
  DFF26/1 -> OR26/1
  DFF26/2 -> T26/1
  OR27/1 -> DFF26/1
  DFF25/1 -> OR25/1
  DFF25/2 -> T25/1
  OR26/1 -> DFF25/1
  DFF24/1 -> OR24/1
  DFF24/2 -> T24/1
  OR25/1 -> DFF24/1
  DFF23/1 -> OR23/1
  DFF23/2 -> T23/1
  OR24/1 -> DFF23/1
  DFF22/1 -> OR22/1
  DFF22/2 -> T22/1
  OR23/1 -> DFF22/1
  DFF21/1 -> OR21/1
  DFF21/2 -> T21/1
  OR22/1 -> DFF21/1
  AND22/1 -> OR22/2
  AND21/1 -> OR21/2
  AND23/1 -> OR23/2
  AND24/1 -> OR24/2
  AND25/1 -> OR25/2
  AND26/1 -> OR26/2
  AND27/1 -> OR27/2
  X16/1 -> AND16/1
  X14/1 -> AND14/1
  X19/1 -> AND19/1
  X18/1 -> AND18/1
  X17/1 -> AND17/1
  X15/1 -> AND15/1
  X20/1 -> AND20/1
  DFF20/1 -> OR20/1
  DFF20/2 -> T20/1
  DFF19/1 -> OR19/1
  DFF19/2 -> T19/1
  OR20/1 -> DFF19/1
  DFF18/1 -> OR18/1
  DFF18/2 -> T18/1
  OR19/1 -> DFF18/1
  DFF17/1 -> OR17/1
  DFF17/2 -> T17/1
  OR18/1 -> DFF17/1
  DFF16/1 -> OR16/1
  DFF16/2 -> T16/1
  OR17/1 -> DFF16/1
  DFF15/1 -> OR15/1
  DFF15/2 -> T15/1
  OR16/1 -> DFF15/1
  DFF14/1 -> OR14/1
  DFF14/2 -> T14/1
  OR15/1 -> DFF14/1
  AND15/1 -> OR15/2
  AND14/1 -> OR14/2
  AND16/1 -> OR16/2
  AND17/1 -> OR17/2
  AND18/1 -> OR18/2
  AND19/1 -> OR19/2
  AND20/1 -> OR20/2
  X9/1 -> AND9/1
  X7/1 -> AND7/1
  X12/1 -> AND12/1
  X11/1 -> AND11/1
  X10/1 -> AND10/1
  X8/1 -> AND8/1
  X13/1 -> AND13/1
  DFF13/1 -> OR13/1
  DFF13/2 -> T13/1
  DFF12/1 -> OR12/1
  DFF12/2 -> T12/1
  OR13/1 -> DFF12/1
  DFF11/1 -> OR11/1
  DFF11/2 -> T11/1
  OR12/1 -> DFF11/1
  DFF10/1 -> OR10/1
  DFF10/2 -> T10/1
  OR11/1 -> DFF10/1
  DFF9/1 -> OR9/1
  DFF9/2 -> T9/1
  OR10/1 -> DFF9/1
  DFF8/1 -> OR8/1
  DFF8/2 -> T8/1
  OR9/1 -> DFF8/1
  DFF7/1 -> OR7/1
  DFF7/2 -> T7/1
  OR8/1 -> DFF7/1
  AND8/1 -> OR8/2
  AND7/1 -> OR7/2
  AND9/1 -> OR9/2
  AND10/1 -> OR10/2
  AND11/1 -> OR11/2
  AND12/1 -> OR12/2
  AND13/1 -> OR13/2
  X2/1 -> AND2/1
  X0/1 -> AND0/1
  X5/1 -> AND5/1
  X4/1 -> AND4/1
  X3/1 -> AND3/1
  X1/1 -> AND1/1
  X6/1 -> AND6/1
  DFF6/1 -> OR6/1
  DFF6/2 -> T6/1
  DFF5/1 -> OR5/1
  DFF5/2 -> T5/1
  OR6/1 -> DFF5/1
  DFF4/1 -> OR4/1
  DFF4/2 -> T4/1
  OR5/1 -> DFF4/1
  DFF3/1 -> OR3/1
  DFF3/2 -> T3/1
  OR4/1 -> DFF3/1
  DFF2/1 -> OR2/1
  DFF2/2 -> T2/1
  OR3/1 -> Logical Operator1/2, DFF2/1
  DFF1/1 -> OR1/1
  DFF1/2 -> T1/1
  OR2/1 -> DFF1/1
  DFF0/1 -> OR0/1
  DFF0/2 -> T0/1
  OR1/1 -> DFF0/1
  OR0/1 -> Data Type Conversion/1, Logical Operator1/1
  AND1/1 -> OR1/2
  AND0/1 -> OR0/2
  AND2/1 -> OR2/2
  AND3/1 -> OR3/2
  AND4/1 -> OR4/2
  AND5/1 -> OR5/2
  AND6/1 -> OR6/2

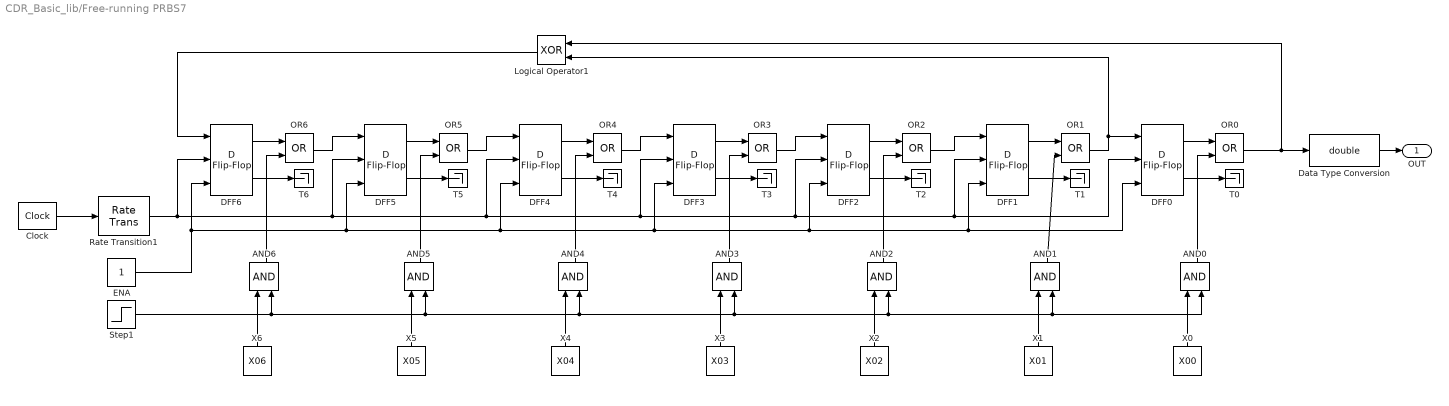
== system CDR_Basic_lib/Free-running PRBS7 ==
  AND{0..6} (7 alike) : Logic  AllPortsSameDT=off  OutDataTypeStr=boolean
  Clock : simulink_extras/Flip Flops/Clock  period=symbol_prd
  DFF{0..6} (7 alike) : simulink_extras/Flip Flops/D Flip-Flop
  Data Type Conversion : DataTypeConversion  OutDataTypeStr=double
  ENA : Constant  OutDataTypeStr=boolean  SampleTime=sample_prd
  Logical Operator1 : Logic  Operator=XOR  AllPortsSameDT=off  OutDataTypeStr=boolean
  OR{0..6} (7 alike) : Logic  Operator=OR  AllPortsSameDT=off  OutDataTypeStr=boolean
  Rate Transition1 : RateTransition  OutPortSampleTime=sample_prd
  Step1 : Step  Time=symbol_prd  Before=1  After=0  SampleTime=sample_prd
  T{0..6} (7 alike) : Terminator
  X0 : Constant  Value=X00  OutDataTypeStr=boolean  SampleTime=sample_prd
  X1 : Constant  Value=X01  OutDataTypeStr=boolean  SampleTime=sample_prd
  X2 : Constant  Value=X02  OutDataTypeStr=boolean  SampleTime=sample_prd
  X3 : Constant  Value=X03  OutDataTypeStr=boolean  SampleTime=sample_prd
  X4 : Constant  Value=X04  OutDataTypeStr=boolean  SampleTime=sample_prd
  X5 : Constant  Value=X05  OutDataTypeStr=boolean  SampleTime=sample_prd
  X6 : Constant  Value=X06  OutDataTypeStr=boolean  SampleTime=sample_prd
  OUT : Outport
  wires:
  Data Type Conversion/1 -> OUT/1
  Rate Transition1/1 -> DFF6/2, DFF5/2, DFF3/2, DFF2/2, DFF1/2, DFF0/2, DFF4/2
  ENA/1 -> DFF5/3, DFF1/3, DFF0/3, DFF2/3, DFF3/3, DFF4/3, DFF6/3
  Clock/1 -> Rate Transition1/1
  X2/1 -> AND2/1
  Step1/1 -> AND0/2, AND1/2, AND2/2, AND3/2, AND4/2, AND5/2, AND6/2
  X0/1 -> AND0/1
  X5/1 -> AND5/1
  X4/1 -> AND4/1
  X3/1 -> AND3/1
  X1/1 -> AND1/1
  X6/1 -> AND6/1
  DFF6/1 -> OR6/1
  DFF6/2 -> T6/1
  DFF5/1 -> OR5/1
  DFF5/2 -> T5/1
  OR6/1 -> DFF5/1
  DFF4/1 -> OR4/1
  DFF4/2 -> T4/1
  OR5/1 -> DFF4/1
  DFF3/1 -> OR3/1
  DFF3/2 -> T3/1
  OR4/1 -> DFF3/1
  DFF2/1 -> OR2/1
  DFF2/2 -> T2/1
  OR3/1 -> DFF2/1
  DFF1/1 -> OR1/1
  DFF1/2 -> T1/1
  OR2/1 -> DFF1/1
  DFF0/1 -> OR0/1
  DFF0/2 -> T0/1
  OR1/1 -> Logical Operator1/2, DFF0/1
  OR0/1 -> Data Type Conversion/1, Logical Operator1/1
  Logical Operator1/1 -> DFF6/1
  AND1/1 -> OR1/2
  AND0/1 -> OR0/2
  AND2/1 -> OR2/2
  AND3/1 -> OR3/2
  AND4/1 -> OR4/2
  AND5/1 -> OR5/2
  AND6/1 -> OR6/2

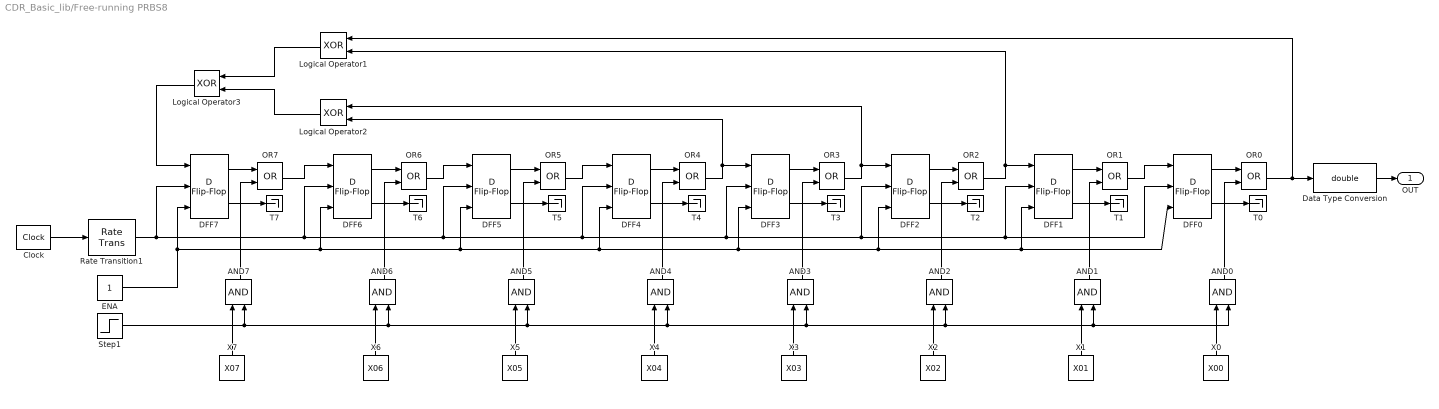
== system CDR_Basic_lib/Free-running PRBS8 ==
  AND{0..7} (8 alike) : Logic  AllPortsSameDT=off  OutDataTypeStr=boolean
  Clock : simulink_extras/Flip Flops/Clock  period=symbol_prd
  DFF{0..7} (8 alike) : simulink_extras/Flip Flops/D Flip-Flop
  Data Type Conversion : DataTypeConversion  OutDataTypeStr=double
  ENA : Constant  OutDataTypeStr=boolean  SampleTime=sample_prd
  Logical Operator1 : Logic  Operator=XOR  AllPortsSameDT=off  OutDataTypeStr=boolean
  Logical Operator2 : Logic  Operator=XOR  AllPortsSameDT=off  OutDataTypeStr=boolean
  Logical Operator3 : Logic  Operator=XOR  AllPortsSameDT=off  OutDataTypeStr=boolean
  OR{0..7} (8 alike) : Logic  Operator=OR  AllPortsSameDT=off  OutDataTypeStr=boolean
  Rate Transition1 : RateTransition  OutPortSampleTime=sample_prd
  Step1 : Step  Time=symbol_prd  Before=1  After=0  SampleTime=sample_prd
  T{0..7} (8 alike) : Terminator
  X0 : Constant  Value=X00  OutDataTypeStr=boolean  SampleTime=sample_prd
  X1 : Constant  Value=X01  OutDataTypeStr=boolean  SampleTime=sample_prd
  X2 : Constant  Value=X02  OutDataTypeStr=boolean  SampleTime=sample_prd
  X3 : Constant  Value=X03  OutDataTypeStr=boolean  SampleTime=sample_prd
  X4 : Constant  Value=X04  OutDataTypeStr=boolean  SampleTime=sample_prd
  X5 : Constant  Value=X05  OutDataTypeStr=boolean  SampleTime=sample_prd
  X6 : Constant  Value=X06  OutDataTypeStr=boolean  SampleTime=sample_prd
  X7 : Constant  Value=X07  OutDataTypeStr=boolean  SampleTime=sample_prd
  OUT : Outport
  wires:
  Data Type Conversion/1 -> OUT/1
  Logical Operator2/1 -> Logical Operator3/2
  Logical Operator1/1 -> Logical Operator3/1
  Logical Operator3/1 -> DFF7/1
  Step1/1 -> AND0/2, AND1/2, AND2/2, AND3/2, AND4/2, AND5/2, AND6/2, AND7/2
  ENA/1 -> DFF3/3, DFF2/3, DFF1/3, DFF0/3, DFF4/3, DFF5/3, DFF6/3, DFF7/3
  Rate Transition1/1 -> DFF4/2, DFF2/2, DFF1/2, DFF0/2, DFF3/2, DFF5/2, DFF6/2, DFF7/2
  OR7/1 -> DFF6/1
  Clock/1 -> Rate Transition1/1
  X7/1 -> AND7/1
  DFF7/1 -> OR7/1
  DFF7/2 -> T7/1
  AND7/1 -> OR7/2
  X2/1 -> AND2/1
  X0/1 -> AND0/1
  X5/1 -> AND5/1
  X4/1 -> AND4/1
  X3/1 -> AND3/1
  X1/1 -> AND1/1
  X6/1 -> AND6/1
  DFF6/1 -> OR6/1
  DFF6/2 -> T6/1
  DFF5/1 -> OR5/1
  DFF5/2 -> T5/1
  OR6/1 -> DFF5/1
  DFF4/1 -> OR4/1
  DFF4/2 -> T4/1
  OR5/1 -> DFF4/1
  DFF3/1 -> OR3/1
  DFF3/2 -> T3/1
  OR4/1 -> Logical Operator2/2, DFF3/1
  DFF2/1 -> OR2/1
  DFF2/2 -> T2/1
  OR3/1 -> Logical Operator2/1, DFF2/1
  DFF1/1 -> OR1/1
  DFF1/2 -> T1/1
  OR2/1 -> Logical Operator1/2, DFF1/1
  DFF0/1 -> OR0/1
  DFF0/2 -> T0/1
  OR1/1 -> DFF0/1
  OR0/1 -> Data Type Conversion/1, Logical Operator1/1
  AND1/1 -> OR1/2
  AND0/1 -> OR0/2
  AND2/1 -> OR2/2
  AND3/1 -> OR3/2
  AND4/1 -> OR4/2
  AND5/1 -> OR5/2
  AND6/1 -> OR6/2

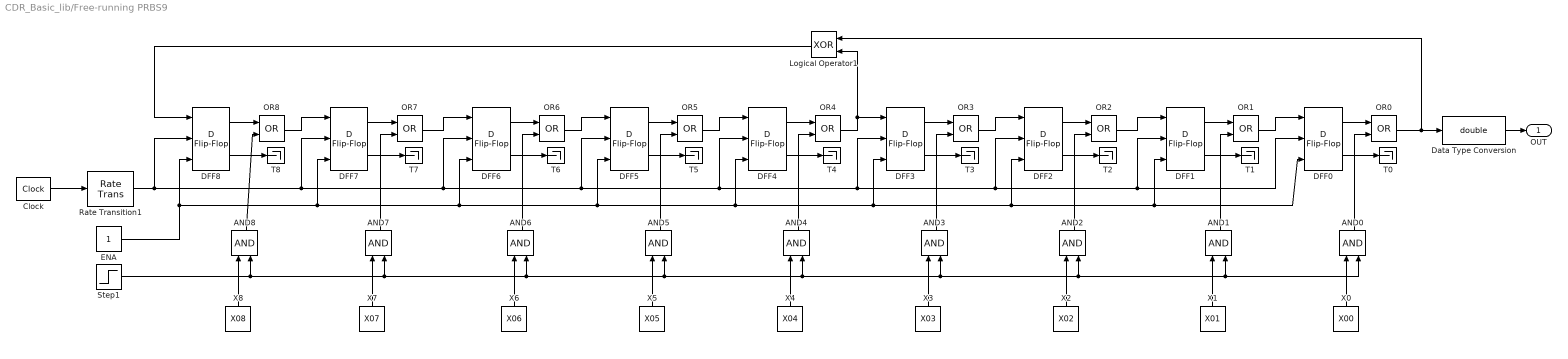
== system CDR_Basic_lib/Free-running PRBS9 ==
  AND{0..8} (9 alike) : Logic  AllPortsSameDT=off  OutDataTypeStr=boolean
  Clock : simulink_extras/Flip Flops/Clock  period=symbol_prd
  DFF{0..8} (9 alike) : simulink_extras/Flip Flops/D Flip-Flop
  Data Type Conversion : DataTypeConversion  OutDataTypeStr=double
  ENA : Constant  OutDataTypeStr=boolean  SampleTime=sample_prd
  Logical Operator1 : Logic  Operator=XOR  AllPortsSameDT=off  OutDataTypeStr=boolean
  OR{0..8} (9 alike) : Logic  Operator=OR  AllPortsSameDT=off  OutDataTypeStr=boolean
  Rate Transition1 : RateTransition  OutPortSampleTime=sample_prd
  Step1 : Step  Time=symbol_prd  Before=1  After=0  SampleTime=sample_prd
  T{0..8} (9 alike) : Terminator
  X0 : Constant  Value=X00  OutDataTypeStr=boolean  SampleTime=sample_prd
  X1 : Constant  Value=X01  OutDataTypeStr=boolean  SampleTime=sample_prd
  X2 : Constant  Value=X02  OutDataTypeStr=boolean  SampleTime=sample_prd
  X3 : Constant  Value=X03  OutDataTypeStr=boolean  SampleTime=sample_prd
  X4 : Constant  Value=X04  OutDataTypeStr=boolean  SampleTime=sample_prd
  X5 : Constant  Value=X05  OutDataTypeStr=boolean  SampleTime=sample_prd
  X6 : Constant  Value=X06  OutDataTypeStr=boolean  SampleTime=sample_prd
  X7 : Constant  Value=X07  OutDataTypeStr=boolean  SampleTime=sample_prd
  X8 : Constant  Value=X08  OutDataTypeStr=boolean  SampleTime=sample_prd
  OUT : Outport
  wires:
  Data Type Conversion/1 -> OUT/1
  Logical Operator1/1 -> DFF8/1
  ENA/1 -> DFF7/3, DFF6/3, DFF5/3, DFF4/3, DFF3/3, DFF2/3, DFF1/3, DFF0/3, DFF8/3
  Rate Transition1/1 -> DFF5/2, DFF4/2, DFF3/2, DFF2/2, DFF1/2, DFF0/2, DFF6/2, DFF7/2, DFF8/2
  OR7/1 -> DFF6/1
  Step1/1 -> AND3/2, AND2/2, AND1/2, AND0/2, AND4/2, AND5/2, AND6/2, AND7/2, AND8/2
  Clock/1 -> Rate Transition1/1
  X7/1 -> AND7/1
  X8/1 -> AND8/1
  DFF8/1 -> OR8/1
  DFF8/2 -> T8/1
  DFF7/1 -> OR7/1
  DFF7/2 -> T7/1
  OR8/1 -> DFF7/1
  AND8/1 -> OR8/2
  AND7/1 -> OR7/2
  X2/1 -> AND2/1
  X0/1 -> AND0/1
  X5/1 -> AND5/1
  X4/1 -> AND4/1
  X3/1 -> AND3/1
  X1/1 -> AND1/1
  X6/1 -> AND6/1
  DFF6/1 -> OR6/1
  DFF6/2 -> T6/1
  DFF5/1 -> OR5/1
  DFF5/2 -> T5/1
  OR6/1 -> DFF5/1
  DFF4/1 -> OR4/1
  DFF4/2 -> T4/1
  OR5/1 -> DFF4/1
  DFF3/1 -> OR3/1
  DFF3/2 -> T3/1
  OR4/1 -> Logical Operator1/2, DFF3/1
  DFF2/1 -> OR2/1
  DFF2/2 -> T2/1
  OR3/1 -> DFF2/1
  DFF1/1 -> OR1/1
  DFF1/2 -> T1/1
  OR2/1 -> DFF1/1
  DFF0/1 -> OR0/1
  DFF0/2 -> T0/1
  OR1/1 -> DFF0/1
  OR0/1 -> Data Type Conversion/1, Logical Operator1/1
  AND1/1 -> OR1/2
  AND0/1 -> OR0/2
  AND2/1 -> OR2/2
  AND3/1 -> OR3/2
  AND4/1 -> OR4/2
  AND5/1 -> OR5/2
  AND6/1 -> OR6/2

== system CDR_Basic_lib/InterfacePDBB ==
  EqualizedData : Inport
  Clock : Inport  Port=2
  RetimedData : Inport  Port=3
  DFEInterface : Inport  Port=4
  DFF2 : Subsystem  mask{DataHigh=VDD, DataLow=0, FF_Threshold=VDD/2}
      mask prompts: DataHigh "High Data Value"; DataLow "Low Data Value"; FF_Threshold "Flip-Flop Threshold"
  DFF3 : Subsystem  mask{DataHigh=VDD, DataLow=0, FF_Threshold=VDD/2}
      mask prompts: DataHigh "High Data Value"; DataLow "Low Data Value"; FF_Threshold "Flip-Flop Threshold"
  Data Type Conversion : DataTypeConversion  OutDataTypeStr=double
  Data Type Conversion1 : DataTypeConversion  OutDataTypeStr=double
  Logical Operator : Logic  Operator=NOT  AllPortsSameDT=off
  Logical Operator1 : Logic  Operator=XOR  AllPortsSameDT=off
  Logical Operator2 : Logic  Operator=XOR  AllPortsSameDT=off
  Y : Outport
  X : Outport  Port=2
  wires:
  DFF3/1(Q) -> DFF2/1(D)
  DFF2/1(Q) -> Logical Operator1/2, Logical Operator2/2
  Logical Operator/1 -> DFF3/Trigger
  Logical Operator2/1 -> Data Type Conversion/1
  Data Type Conversion/1 -> Y/1
  Logical Operator1/1 -> Data Type Conversion1/1
  Data Type Conversion1/1 -> X/1
  EqualizedData/1 -> DFF3/1(D)
  Clock/1 -> Logical Operator/1, DFF2/Trigger
  RetimedData/1 -> Logical Operator2/1
  DFEInterface/1 -> Logical Operator1/1

== system CDR_Basic_lib/Mux ==
  a : Inport
  sel : Inport  Port=2
  b : Inport  Port=3
  Switch : Switch  Threshold=MuxThreshold
  out : Outport
  wires:
  sel/1 -> Switch/2
  b/1 -> Switch/3
  a/1 -> Switch/1
  Switch/1 -> out/1

== system CDR_Basic_lib/PDBB ==
  EqualizedData : Inport
  Clock : Inport  Port=2
  DFF1 : Subsystem  mask{DataHigh=VDD, DataLow=0, FF_Threshold=VDD/2}
      mask prompts: DataHigh "High Data Value"; DataLow "Low Data Value"; FF_Threshold "Flip-Flop Threshold"
  DFF2 : Subsystem  mask{DataHigh=VDD, DataLow=0, FF_Threshold=VDD/2}
      mask prompts: DataHigh "High Data Value"; DataLow "Low Data Value"; FF_Threshold "Flip-Flop Threshold"
  DFF3 : Subsystem  mask{DataHigh=VDD, DataLow=0, FF_Threshold=VDD/2}
      mask prompts: DataHigh "High Data Value"; DataLow "Low Data Value"; FF_Threshold "Flip-Flop Threshold"
  DFF5 : Subsystem  mask{DataHigh=VDD, DataLow=0, FF_Threshold=VDD/2}
      mask prompts: DataHigh "High Data Value"; DataLow "Low Data Value"; FF_Threshold "Flip-Flop Threshold"
  Data Type Conversion : DataTypeConversion  OutDataTypeStr=double
  Data Type Conversion1 : DataTypeConversion  OutDataTypeStr=double
  Logical Operator : Logic  Operator=NOT  AllPortsSameDT=off
  Logical Operator1 : Logic  Operator=XOR  AllPortsSameDT=off
  Logical Operator2 : Logic  Operator=XOR  AllPortsSameDT=off
  Early : Outport
  Late : Outport  Port=2
  RetimedData : Outport  Port=3
  wires:
  DFF3/1(Q) -> DFF2/1(D)
  DFF5/1(Q) -> Logical Operator2/1, RetimedData/1, DFF1/1(D)
  DFF2/1(Q) -> Logical Operator1/2, Logical Operator2/2
  DFF1/1(Q) -> Logical Operator1/1
  Logical Operator/1 -> DFF3/Trigger
  Logical Operator2/1 -> Data Type Conversion/1
  Data Type Conversion/1 -> Early/1
  Logical Operator1/1 -> Data Type Conversion1/1
  Data Type Conversion1/1 -> Late/1
  EqualizedData/1 -> DFF5/1(D), DFF3/1(D)
  Clock/1 -> Logical Operator/1, DFF5/Trigger, DFF1/Trigger, DFF2/Trigger

== system CDR_Basic_lib/Phase Interpolator ==
  note: Phase select introduces a phase offset
  VCO Phase : Inport
  Phase Shift : Inport  Port=2
  3 : Constant  Value=2*pi
  7 : Math  Operator=mod  SaturateOnIntegerOverflow=on
  Fcn : Fcn  SampleTime=Ts
  Fcn1 : Fcn  Expr=cos(u[1])  SampleTime=Ts
  Fcn2 : Fcn  Expr=cos(u[1] - 0.785398)  SampleTime=Ts
  Fcn3 : Fcn  Expr=sin(u[1] - 0.785398)  SampleTime=Ts
  Sum : Sum  SaturateOnIntegerOverflow=on  InputSameDT=on  OutDataTypeStr=Inherit: Same as first input
  Sum1 : Sum  Inputs=|++  SaturateOnIntegerOverflow=on  InputSameDT=on  OutDataTypeStr=Inherit: Same as first input
  0 deg : Outport
  -45 deg : Outport  Port=2
  -90 deg : Outport  Port=3
  -135 deg : Outport  Port=4
  Phi : Outport  Port=5
  wires:
  7/1 -> Fcn1/1, Fcn2/1, Fcn/1, Fcn3/1, Phi/1  "Phase"
  Sum/1 -> 7/1
  Phase Shift/1 -> Sum1/2
  VCO Phase/1 -> Sum1/1
  Fcn/1 -> -90 deg/1
  Fcn1/1 -> 0 deg/1
  3/1 -> Sum/2, 7/2
  Fcn2/1 -> -45 deg/1
  Fcn3/1 -> -135 deg/1
  Sum1/1 -> Sum/1

== system CDR_Basic_lib/Quad PI ==
  note: Phase Shift introduces a phase offset
      | Q ph err introduces a quadrature phase error
  VCO Phase : Inport
  Phase Shift : Inport  Port=2
  Q ph err : Inport  Port=3
  3 : Constant  Value=2*pi
  7 : Math  Operator=mod  SaturateOnIntegerOverflow=on
  Fcn1 : Fcn  SampleTime=Ts
  Fcn2 : Fcn  Expr=-cos(u[1])  SampleTime=Ts
  Sum : Sum  SaturateOnIntegerOverflow=on  InputSameDT=on  OutDataTypeStr=Inherit: Same as first input
  Sum1 : Sum  Inputs=|++  SaturateOnIntegerOverflow=on  InputSameDT=on  OutDataTypeStr=Inherit: Same as first input
  Sum2 : Sum  SaturateOnIntegerOverflow=on  InputSameDT=on  OutDataTypeStr=Inherit: Same as first input
  I-0 : Outport
  Q-90 : Outport  Port=2
  Phi : Outport  Port=3
  wires:
  Sum1/1 -> Sum/1
  Fcn2/1 -> Q-90/1
  3/1 -> 7/2, Sum/2
  Fcn1/1 -> I-0/1
  VCO Phase/1 -> Sum1/1
  Phase Shift/1 -> Sum1/2
  Sum/1 -> 7/1
  7/1 -> Fcn1/1, Sum2/1, Phi/1  "Phase"
  Sum2/1 -> Fcn2/1
  Q ph err/1 -> Sum2/2

== system CDR_Basic_lib/S & H ==
  S : Inport
  Trigger : TriggerPort
  H : Outport
  wires:
  S/1 -> H/1
